simulink model "bioreactor"  (R2013a)
settings: Solver=ode23  StartTime=0.0  StopTime=100  RelTol=1e-3
values from neighbouring files (symbols this model uses):
  alpha = 2.2    [bio_modelling_parameters.m]
  beta = 0.2    [bio_modelling_parameters.m]
  Yxs = 0.4    [bio_modelling_parameters.m]
undefined symbols (not defined in the file or in its folder): D, miu, P, S, Sf, X
settings Model: Creator=sayan  LastModifiedBy=Dibyashree

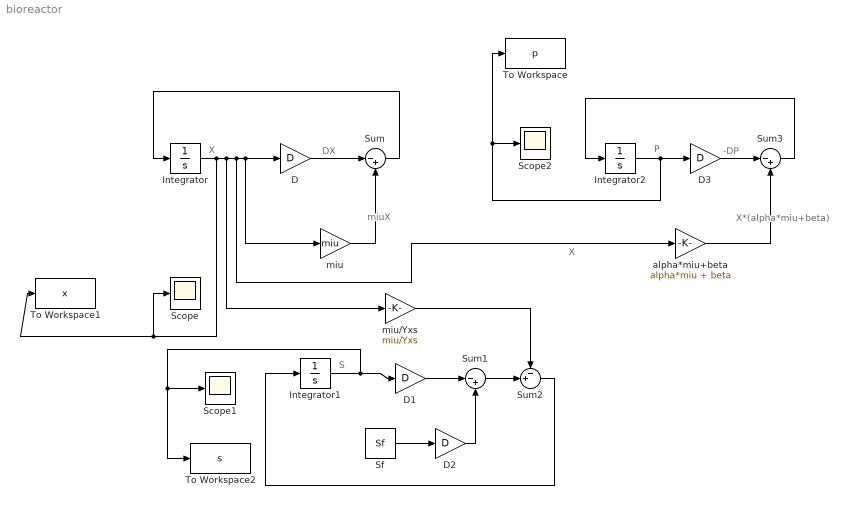
== system bioreactor ==
  note: -DP
  note: X*(alpha*miu+beta)
  note: X
  note: P
  note: miuX
  note: DX
  note: X
  note: S
  D{,1..3} (4 alike) : Gain  Gain=D
  Integrator : Integrator  InitialCondition=X
  Integrator1 : Integrator  InitialCondition=S
  Integrator2 : Integrator  InitialCondition=P
  Scope : Scope
  Scope1 : Scope
  Scope2 : Scope
      settings: TimeRange=20  YMin=5  YMax=25  SaveName=ScopeData2
  Sf : Constant  Value=Sf
  Sum : Sum  Inputs=|-+
  Sum1 : Sum  Inputs=|-+
  Sum2 : Sum  Inputs=-+|
  Sum3 : Sum  Inputs=|-+
  To Workspace : ToWorkspace  VariableName=p  SampleTime=-1  SaveFormat=Timeseries
  To Workspace1 : ToWorkspace  VariableName=x  SampleTime=-1  SaveFormat=Timeseries
  To Workspace2 : ToWorkspace  VariableName=s  SampleTime=-1  SaveFormat=Timeseries
  alpha*miu+beta : Gain  Gain=alpha*miu + beta
  miu : Gain  Gain=miu
  miu/Yxs : Gain  Gain=miu/Yxs
  wires:
  Integrator/1 -> To Workspace1/1, Scope/1, miu/Yxs/1, alpha*miu+beta/1, miu/1, D/1
  D/1 -> Sum/1
  miu/1 -> Sum/2
  Sum/1 -> Integrator/1
  Integrator1/1 -> To Workspace2/1, Scope1/1, D1/1
  D1/1 -> Sum1/1
  Sf/1 -> D2/1
  D2/1 -> Sum1/2
  Sum1/1 -> Sum2/2
  miu/Yxs/1 -> Sum2/1
  Sum2/1 -> Integrator1/1
  Integrator2/1 -> To Workspace/1, Scope2/1, D3/1
  D3/1 -> Sum3/1
  alpha*miu+beta/1 -> Sum3/2
  Sum3/1 -> Integrator2/1
